simulink model "MyEngine_RTW"  (Simulink 10.3)
settings: Solver=ode1  StartTime=0.0  StopTime=inf  FixedStep=0.0002  RelTol=1e-3
PreLoadFcn:
  | vehicle = 'Car'; if ~length(which('cmcmd')), cmenv; end
  | MyEngine_RTW_bus
InitFcn:
  | vehicle = 'Car'; if ~length(which('cmcmd')), cmenv; end
  | MyEngine_RTW_bus
libraries: simulink x2, CarMaker4SL x2
Description:
  | CarMaker Plug-in Model Target
settings Model: Creator=ml  ModifiedByFormat=IPG  LastModifiedBy=IPG  MultithreadedSim=on
settings DataIOCC: LimitDataPoints=on
settings DebuggingCC: SFExecutionAtInitializationDiag=warning
settings HardwareCC: TargetHWDeviceType=32-bit Generic  ProdEqTarget=off
settings RTWCC: Description=CarMaker Plug-in Model Target  SystemTargetFile=CarMaker.tlc  TemplateMakefile=CarMaker_unix-win64.tmf
settings CodeAppCC: MaxIdLength=63
settings STFCustomTargetCC: ModelReferenceCompliant=off  CodeInterfacePackaging=Reusable function  CPPClassGenCompliant=on  GRTInterface=off  GenerateAllocFcn=on  SystemTargetFile=CarMaker.tlc
settings GRTTargetCC: ModelReferenceCompliant=off  ParMdlRefBuildCompliant=off  CompOptLevelCompliant=off  ConcurrentExecutionCompliant=off  MatFileLogging=off  CodeInterfacePackaging=Reusable function  GRTInterface=off  GenerateAllocFcn=on  UseToolchainInfoCompliant=off  ExtModeMexFile=noextcomm
settings CustomProperty: DataType=string
settings EnumStrPairs: String=Car

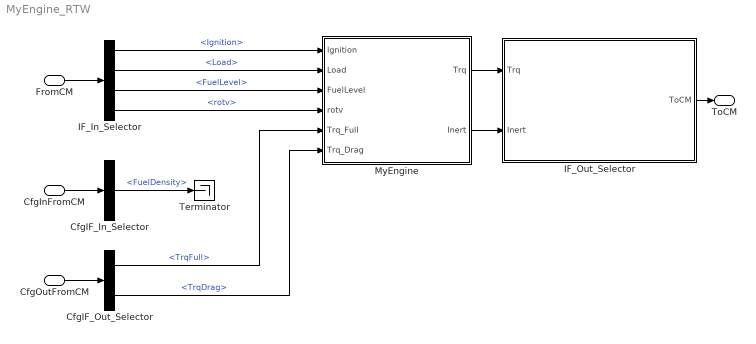
== system MyEngine_RTW ==
  FromCM : Inport  OutDataTypeStr=Bus: cmPTEngineIn
  CfgInFromCM : Inport  Port=2  OutDataTypeStr=Bus: cmPTEngineCfgIn
  CfgOutFromCM : Inport  Port=3  OutDataTypeStr=Bus: cmPTEngineCfgOut
  CfgIF_In_Selector : BusSelector  OutputSignals=FuelDensity
  CfgIF_Out_Selector : BusSelector  OutputSignals=TrqFull,TrqDrag
  IF_In_Selector : BusSelector  OutputSignals=Ignition,Load,FuelLevel,rotv
  IF_Out_Selector : Subsystem  mask(Signal Selection){}
      mask help: Signal Selection Block
      settings: OpenFcn=cmSignalSelect('SignalSelection_CB',gcb)
  MyEngine : Subsystem
  Terminator : Terminator
  ToCM : Outport  OutDataTypeStr=Bus: cmPTEngineOut  VectorParamsAs1DForOutWhenUnconnected=off
  wires:
  FromCM/1 -> IF_In_Selector/1
  IF_Out_Selector/1(ToCM) -> ToCM/1
  CfgInFromCM/1 -> CfgIF_In_Selector/1
  CfgOutFromCM/1 -> CfgIF_Out_Selector/1
  IF_In_Selector/1 -> MyEngine/1(Ignition)  "<Ignition>"
  IF_In_Selector/2 -> MyEngine/2(Load)  "<Load>"
  IF_In_Selector/3 -> MyEngine/3(FuelLevel)  "<FuelLevel>"
  IF_In_Selector/4 -> MyEngine/4(rotv)  "<rotv>"
  CfgIF_Out_Selector/1 -> MyEngine/5(Trq_Full)  "<TrqFull>"
  CfgIF_Out_Selector/2 -> MyEngine/6(Trq_Drag)  "<TrqDrag>"
  MyEngine/2(Inert) -> IF_Out_Selector/2(Inert)
  MyEngine/1(Trq) -> IF_Out_Selector/1(Trq)
  CfgIF_In_Selector/1 -> Terminator/1  "<FuelDensity>"

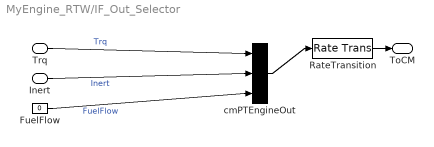
== system MyEngine_RTW/IF_Out_Selector ==
  Trq : Inport
  Inert : Inport  Port=2
  FuelFlow : Constant  Value=0
  RateTransition : RateTransition  OutPortSampleTime=str2num(get_param(bdroot,'FixedStep'))
  cmPTEngineOut : BusCreator  Inputs=3
  ToCM : Outport  VectorParamsAs1DForOutWhenUnconnected=off
  wires:
  RateTransition/1 -> ToCM/1
  cmPTEngineOut/1 -> RateTransition/1
  FuelFlow/1 -> cmPTEngineOut/3  "FuelFlow"
  Trq/1 -> cmPTEngineOut/1  "Trq"
  Inert/1 -> cmPTEngineOut/2  "Inert"

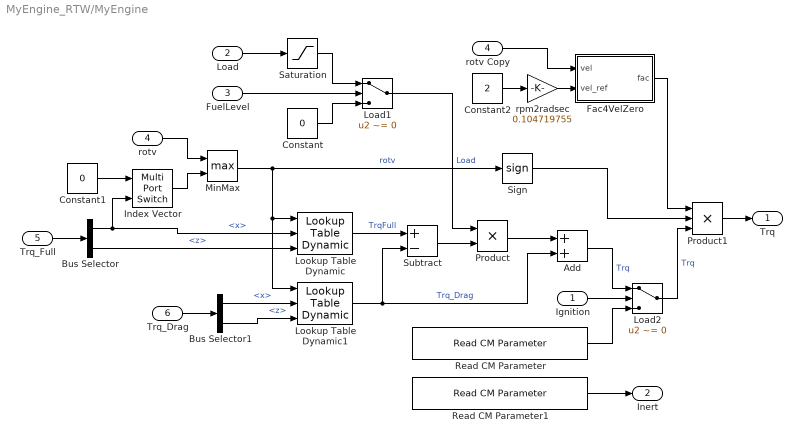
== system MyEngine_RTW/MyEngine ==
  Ignition : Inport
  Load : Inport  Port=2
  FuelLevel : Inport  Port=3
  rotv : Inport  Port=4
  Trq_Full : Inport  Port=5
  Trq_Drag : Inport  Port=6
  Add : Sum
  Bus Selector : BusSelector  OutputSignals=x,z
  Bus Selector1 : BusSelector  OutputSignals=x,z
  Constant : Constant  Value=0
  Constant1 : Constant  Value=0
  Constant2 : Constant  Value=2
  Fac4VelZero : Subsystem
  Index Vector : MultiPortSwitch  DataPortOrder=Zero-based contiguous  Inputs=1  zeroidx=on
  Load1 : Switch  Criteria=u2 ~= 0
  Load2 : Switch  Criteria=u2 ~= 0
  Lookup Table Dynamic : simulink/Lookup Tables/Lookup Table Dynamic  LookUpMeth=Interpolation-Use End Values  OutDataTypeStr=float('double')  OutputDataTypeScalingMode=Specify via dialog  OutDataType=float('double')  OutScaling=2^-10  DoSatur=off
  Lookup Table Dynamic1 : simulink/Lookup Tables/Lookup Table Dynamic  LookUpMeth=Interpolation-Use End Values  OutDataTypeStr=float('double')  OutputDataTypeScalingMode=Specify via dialog  OutDataType=float('double')  OutScaling=2^-10  DoSatur=off
  MinMax : MinMax  Function=max  Inputs=2
  Product : Product  RndMeth=Zero
  Product1 : Product  Inputs=3  RndMeth=Zero
  Read CM Parameter : CarMaker4SL/Read CM Parameter  xfile=Vehicle  xkey=PowerTrain.MyEngine.TrqKl15Off  xnout=1  xdefaults=[]  xmuxed=on
      settings: SourceProductName=CarMaker4SL
  Read CM Parameter1 : CarMaker4SL/Read CM Parameter  xfile=Vehicle  xkey=PowerTrain.Engine.I  xnout=1  xdefaults=0.1  xmuxed=on
      settings: SourceProductName=CarMaker4SL
  Saturation : Saturate  UpperLimit=1  LowerLimit=0
  Sign : Signum
  Subtract : Sum  Inputs=+-
  rotv Copy : InportShadow  Port=4
  rpm2radsec : Gain  Gain=0.104719755
  Trq : Outport  VectorParamsAs1DForOutWhenUnconnected=off
  Inert : Outport  Port=2  VectorParamsAs1DForOutWhenUnconnected=off
  wires:
  Load/1 -> Saturation/1
  FuelLevel/1 -> Load1/2
  Saturation/1 -> Load1/1
  Constant/1 -> Load1/3
  Load1/1 -> Product/1  "Load"
  Ignition/1 -> Load2/2
  Read CM Parameter/1 -> Load2/3
  Read CM Parameter1/1 -> Inert/1
  Trq_Full/1 -> Bus Selector/1
  Bus Selector/1 -> Index Vector/2, Lookup Table Dynamic/2  "<x>"
  Constant1/1 -> Index Vector/1
  Index Vector/1 -> MinMax/2
  MinMax/1 -> Lookup Table Dynamic1/1, Lookup Table Dynamic/1, Sign/1  "rotv"
  Trq_Drag/1 -> Bus Selector1/1
  Bus Selector/2 -> Lookup Table Dynamic/3  "<z>"
  Bus Selector1/1 -> Lookup Table Dynamic1/2  "<x>"
  Bus Selector1/2 -> Lookup Table Dynamic1/3  "<z>"
  Lookup Table Dynamic/1 -> Subtract/1  "TrqFull"
  Lookup Table Dynamic1/1 -> Subtract/2, Add/2  "Trq_Drag"
  Subtract/1 -> Product/2
  Product/1 -> Add/1
  Add/1 -> Load2/1  "Trq"
  Product1/1 -> Trq/1
  Load2/1 -> Product1/3  "Trq"
  Constant2/1 -> rpm2radsec/1
  rpm2radsec/1 -> Fac4VelZero/2(vel_ref)
  rotv Copy/1 -> Fac4VelZero/1(vel)
  Fac4VelZero/1(fac) -> Product1/1
  Sign/1 -> Product1/2
  rotv/1 -> MinMax/1

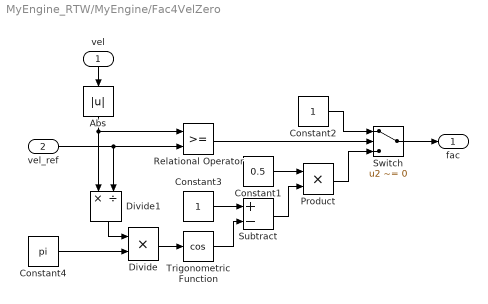
== system MyEngine_RTW/MyEngine/Fac4VelZero ==
  vel : Inport
  vel_ref : Inport  Port=2
  Abs : Abs
  Constant1 : Constant  Value=0.5
  Constant2 : Constant
  Constant3 : Constant
  Constant4 : Constant  Value=pi
  Divide : Product  Inputs=**
  Divide1 : Product  Inputs=*/
  Product : Product  RndMeth=Zero
  Relational Operator : RelationalOperator  OutDataTypeStr=boolean  RndMeth=Nearest
  Subtract : Sum  Inputs=+-
  Switch : Switch  Criteria=u2 ~= 0
  Trigonometric Function : Trigonometry  Operator=cos
  fac : Outport  VectorParamsAs1DForOutWhenUnconnected=off
  wires:
  Abs/1 -> Relational Operator/1, Divide1/1
  Relational Operator/1 -> Switch/2
  Constant2/1 -> Switch/1
  vel/1 -> Abs/1
  Switch/1 -> fac/1
  Product/1 -> Switch/3
  Constant1/1 -> Product/1
  Constant3/1 -> Subtract/1
  Subtract/1 -> Product/2
  Trigonometric Function/1 -> Subtract/2
  Divide/1 -> Trigonometric Function/1
  Constant4/1 -> Divide/2
  vel_ref/1 -> Relational Operator/2, Divide1/2
  Divide1/1 -> Divide/1
